simulink model "simulate_engine_cl"  (R2023b)
settings: Solver=VariableStepAuto  StartTime=0.0  StopTime=100  RelTol=1e-3
libraries: fl_lib x6, nesl_utility x6, simulink x1, ee_lib x1
settings Model: Creator=franc  LastModifiedBy=franc

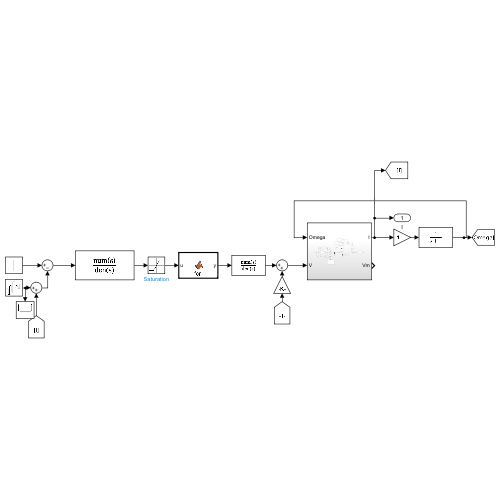
[thumbnail: Simulink's stored preview of the top-level diagram]
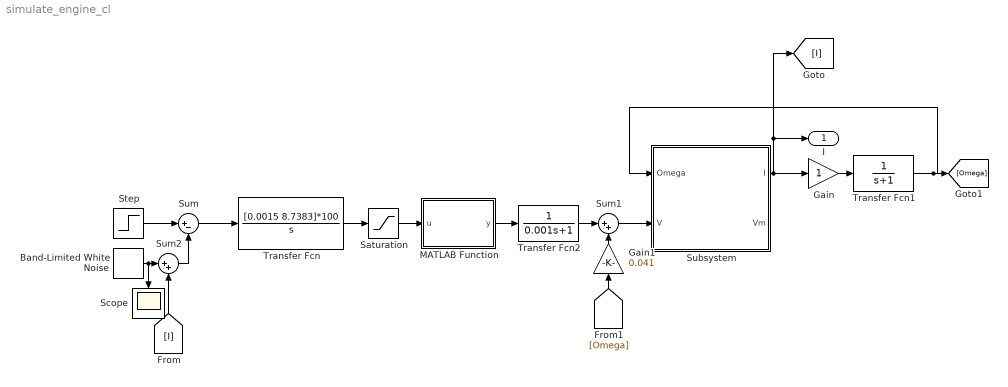
== system simulate_engine_cl ==
  Band-Limited White Noise : simulink/Sources/Band-Limited White Noise  Cov=[1e-4]  Ts=0.1  seed=[23341]
  Gain : Gain
  Gain1 : Gain  Gain=0.041
  MATLAB Function : MATLAB Function  TreatAsAtomicUnit=on
  Saturation : Saturate  UpperLimit=24  LowerLimit=-24
  Scope : Scope
  Step : Step  SampleTime=0
  Subsystem : Subsystem
  Sum : Sum  Inputs=|+-
  Sum1 : Sum  Inputs=|++
  Sum2 : Sum  Inputs=|++
  Transfer Fcn : TransferFcn  Numerator=[0.0015 8.7383]*100  Denominator=[1 0]
  Transfer Fcn1 : TransferFcn  Denominator=[1 1]
  Transfer Fcn2 : TransferFcn  Denominator=[0.001 1]
  I : Outport
  wires:
  Subsystem/1(I) -> Gain/1, [I], I/1
  Step/1 -> Sum/1
  Sum/1 -> Transfer Fcn/1
  Transfer Fcn/1 -> Saturation/1
  Saturation/1 -> MATLAB Function/1(u)
  Transfer Fcn1/1 -> [Omega], Subsystem/1(Omega)
  Gain/1 -> Transfer Fcn1/1
  Sum1/1 -> Subsystem/2(V)
  Gain1/1 -> Sum1/2
  [Omega] -> Gain1/1
  [I] -> Sum2/2
  Sum2/1 -> Sum/2
  Band-Limited White Noise/1 -> Sum2/1, Scope/1
  MATLAB Function/1(y) -> Transfer Fcn2/1
  Transfer Fcn2/1 -> Sum1/1

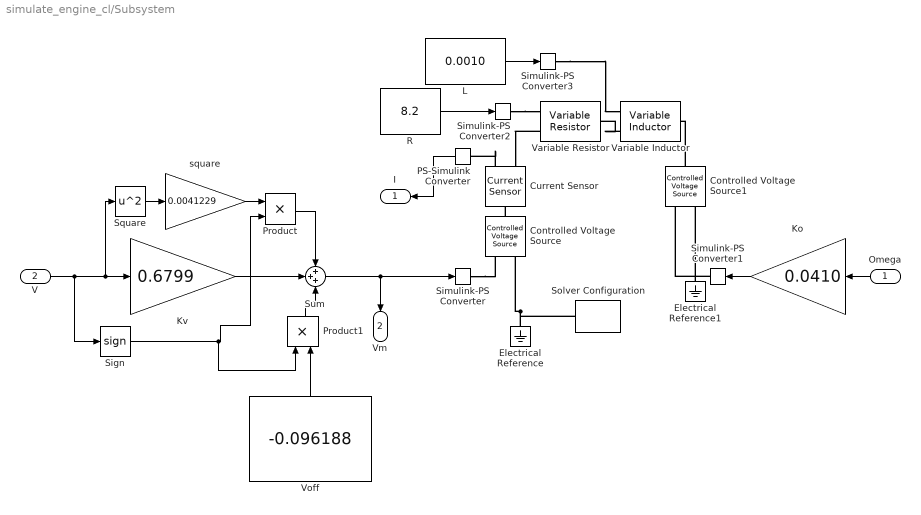
== system simulate_engine_cl/Subsystem ==
  Omega : Inport
  V : Inport  Port=2
  Controlled Voltage Source : fl_lib/Electrical/Electrical Sources/Controlled Voltage Source
  Controlled Voltage Source1 : fl_lib/Electrical/Electrical Sources/Controlled Voltage Source
  Current Sensor : fl_lib/Electrical/Electrical Sensors/Current Sensor
  Electrical Reference : fl_lib/Electrical/Electrical Elements/Electrical Reference
  Electrical Reference1 : fl_lib/Electrical/Electrical Elements/Electrical Reference
  Ko : Gain  Gain=0.0410
  Kv : Gain  Gain=0.6799
  L : Constant  Value=0.0010
  PS-Simulink Converter : nesl_utility/PS-Simulink Converter  PhysicalDomain=network_engine_domain  SubClassName=ps_output  LeftPortType=input  RightPortType=output  PseudoPeriodic=off  Frequencies=[]  VectorFormat=inherit  Unit=inherit  AffineConversion=off
  Product : Product
  Product1 : Product
  R : Constant  Value=8.2
  Sign : Signum
  Simulink-PS Converter{,1..3} (4 alike) : nesl_utility/Simulink-PS Converter  PhysicalDomain=network_engine_domain  SubClassName=ps_input  LeftPortType=input  RightPortType=output  PseudoPeriodic=off  Frequencies=[]  NoiseDistribution=none  NoiseParameters=[]  Unit=1  AffineConversion=off  FilteringAndDerivatives=provide  SimscapeFilterOrder=1  InputFilterTimeConstant=0.001  UdotUserProvided=0
  Solver Configuration : nesl_utility/Solver Configuration  PhysicalDomain=network_engine_domain  SubClassName=solver  LeftPortType=input  RightPortType=generic  Tones=[]  Harmonics=[]  SimulateNoise=off  Profile=off  UseLocalSampling=off  EnableSwitchedLinearOptims=on  FrequencyDomain=off  UseCCode=off  RelTol=0.001  AbsTol=0.001  MinStep=1e-09  ToWorkspace=off  RevertToSquareIcSolve=off  NumHomotopyIterations=100  PhasorMode=off  PhasorModeNumHarmonics=1  ConsistencySolver=NEWTON_XTOL_AFTER_FTOL  IndexReductionMethod=DerivativeReplacement  DoDC=off  ResidualTolerance=1e-09  ConsistencyTolSource=GLOBAL  ConsistencyAbsTol=0.001  ConsistencyRelTol=0.001  ConsistencyTolFactor=0.001  UseLocalSolver=off  LocalSolverChoice=NE_BACKWARD_EULER_ADVANCER  ResolveIndetEquations=on  FunctionEvalNumThread=1  LocalSolverSampleTime=0.001  DoFixedCost=off  MaxNonlinIter=3  MaxModeIter=2  ComputeImpulses=off  ImpulseIterations=2  LinearAlgebra=auto  LinearAlgebraNumThread=0  EquationFormulation=NE_TIME_EF  DelaysMemoryBudget=1024  AutomaticFiltering=on  FilteringTimeConstant=0.001  PartitionStorageMethod=AS_NEEDED  PartitionMemoryBudget=1024  PartitionMethod=ROBUST  MultibodyUseLocalSolver=off  MultibodyLocalSolverChoice=ODE1  MultibodyLocalSolverSampleTime=0.001
  Square : Math  Operator=square
  Sum : Sum  Inputs=+++
  Variable Inductor : ee_lib/Passive/Variable Inductor  prm=1  Lmin=1e-6 H  g=1e-9 1/Ohm  i0=0 A  phi0=0 Wb
      settings: InternalSimscapePortConfiguration="{\"Bottom\":[],\"Left\":[{\"id\":\"L\",\"label\":\"L\",\"type\":\"input\"},{\"id\":\"p\",\"label\":\"+\",\"type\":\"foundation.electrical.electrical\"}],\"Right\":[{\"id\":\"n\",\"label\":\"-\",\"type\":\"foundation.electrical.electrical\"}],\"Top\":[]}"
  Variable Resistor : fl_lib/Electrical/Electrical Elements/Variable Resistor  Rmin=0 Ohm  thermalEnable=false  thermal_mass=1 J/K  i_specify=off  i_priority=None  i=0 A  i_nominal_specify=off  i_nominal_unit=A  i_nominal_value=1  v_specify=off  v_priority=None  v=0 V  v_nominal_specify=off  v_nominal_unit=V  v_nominal_value=1  T_specify=off  T_priority=None  T=300 K  T_nominal_specify=off  T_nominal_unit=K  T_nominal_value=1
  Voff : Constant  Value=-0.096188
  square : Gain  Gain=0.0041229
  I : Outport
  Vm : Outport  Port=2
  wires:
  Product1/1 -> Sum/3
  PS-Simulink Converter/1 -> I/1
  V/1 -> Sign/1, Square/1, Kv/1
  R/1 -> Simulink-PS Converter2/1
  L/1 -> Simulink-PS Converter3/1
  Omega/1 -> Ko/1
  Voff/1 -> Product1/2
  Kv/1 -> Sum/2
  Sum/1 -> Vm/1, Simulink-PS Converter/1
  Square/1 -> square/1
  square/1 -> Product/1
  Sign/1 -> Product1/1, Product/2
  Product/1 -> Sum/1
  Ko/1 -> Simulink-PS Converter1/1
  connections:
  Controlled Voltage Source/LConn1 -- Current Sensor/LConn1
  Simulink-PS Converter3/RConn1 -- Variable Inductor/LConn1
  Controlled Voltage Source1/LConn1 -- Variable Inductor/RConn1
  Current Sensor/RConn1 -- PS-Simulink Converter/LConn1
  Variable Inductor/LConn2 -- Variable Resistor/RConn1
  Simulink-PS Converter1/RConn1 -- Controlled Voltage Source1/RConn1
  Simulink-PS Converter/RConn1 -- Controlled Voltage Source/RConn1
  Simulink-PS Converter2/RConn1 -- Variable Resistor/LConn1
  Variable Resistor/LConn2 -- Current Sensor/RConn2
  Electrical Reference1/LConn1 -- Controlled Voltage Source1/RConn2
  Solver Configuration/RConn1 -- Controlled Voltage Source/RConn2 -- Electrical Reference/LConn1

== matlab function simulate_engine_cl/MATLAB Function ==
  data: u input; y output
function y = fcn(u)

y = Vm2Vb(u);
